simulink model "aero"  (R2024a)
settings: configuration reference "standardSILConfiguraitonParams" (kept outside this file)
undefined symbols (not defined in the file): m2ft, vehicleParams
libraries: aerolibconvert2 x5, aerolibasang x1, matrix_library x1
settings Model: Creator=GTAR  LastModifiedBy=jerem
settings ConfigSetRef: SourceName=standardSILConfiguraitonParams  SourceLocation=Base Workspace

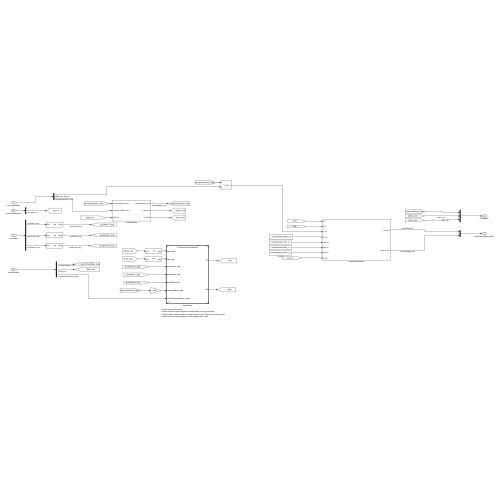
[thumbnail: Simulink's stored preview of the top-level diagram]
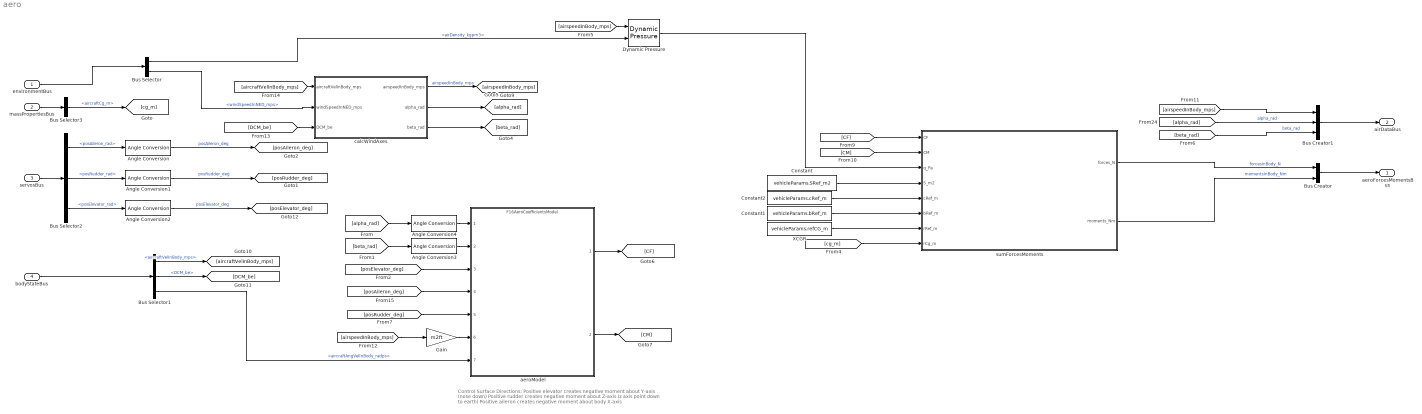
== system aero ==
  note: Control Surface Directions:
      | Positive elevator creates negative moment about Y-axis (nose down)
      | Positive rudder creates negative moment about Z-axis (z axis point down to earth)
      | Positive aileron creates negative moment about body X-axis
  environmentBus : Inport  OutDataTypeStr=Bus: EnvironmentBus
  massPropertiesBus : Inport  Port=2  OutDataTypeStr=Bus: MassPropertiesBus
  servosBus : Inport  Port=3  OutDataTypeStr=Bus: ServosBus
  bodyStateBus : Inport  Port=4  OutDataTypeStr=Bus: BodyStateBus
  Angle Conversion{,1..4} (5 alike) : aerolibconvert2/Angle Conversion  IU=rad  OU=deg
  Bus Creator : BusCreator  Inputs=2
  Bus Creator1 : BusCreator  Inputs=3
  Bus Selector : BusSelector  OutputSignals=AirEnvironment.airDensity_kgpm3,AirEnvironment.windSpeedInNED_mps
  Bus Selector1 : BusSelector  OutputSignals=aircraftVelInBody_mps,DCM_be,aircraftAngVelInBody_radps
  Bus Selector2 : BusSelector  OutputSignals=ServosF16Bus.posAileron_rad,ServosF16Bus.posRudder_rad,ServosF16Bus.posElevator_rad
  Bus Selector3 : BusSelector  OutputSignals=aircraftCg_m
  Constant : Constant  Value=vehicleParams.SRef_m2
  Constant1 : Constant  Value=vehicleParams.bRef_m
  Constant2 : Constant  Value=vehicleParams.cRef_m
  Dynamic Pressure : aerolibasang/Dynamic Pressure
  Gain : Gain  Gain=m2ft
  XCGR : Constant  Value=vehicleParams.refCG_m
  aeroModel : ModelReference  ModelNameDialog=F16AeroCoefficientsModel.slx  SimulationMode=Normal  ModelReferenceVersion=1.183
  calcWindAxes : Subsystem
  sumForcesMoments : Subsystem
  aeroForcesMomentsBus : Outport  OutDataTypeStr=Bus: ComponentForcesMomentsBus
  airDataBus : Outport  Port=2  OutDataTypeStr=Bus: AirData
  wires:
  Bus Creator/1 -> aeroForcesMomentsBus/1
  sumForcesMoments/1(forces_N) -> Bus Creator/1  "forcesInBody_N"
  sumForcesMoments/2(moments_Nm) -> Bus Creator/2  "momentsInBody_Nm"
  [cg_m] -> sumForcesMoments/8(rCg_m)
  Dynamic Pressure/1 -> sumForcesMoments/3(q_Pa)
  Angle Conversion/1 -> [posAileron_deg]  "posAileron_deg"
  environmentBus/1 -> Bus Selector/1
  Bus Selector/1 -> Dynamic Pressure/2  "<airDensity_kgpm3>"
  Bus Selector/2 -> calcWindAxes/2(windSpeedInNED_mps)  "<windSpeedInNED_mps>"
  servosBus/1 -> Bus Selector2/1
  Bus Selector2/1 -> Angle Conversion/1  "<posAileron_rad>"
  massPropertiesBus/1 -> Bus Selector3/1
  Bus Selector3/1 -> [cg_m]  "<aircraftCg_m>"
  bodyStateBus/1 -> Bus Selector1/1
  Bus Creator1/1 -> airDataBus/1
  Bus Selector2/2 -> Angle Conversion1/1  "<posRudder_rad>"
  Bus Selector2/3 -> Angle Conversion2/1  "<posElevator_rad>"
  Angle Conversion1/1 -> [posRudder_deg]  "posRudder_deg"
  Angle Conversion2/1 -> [posElevator_deg]  "posElevator_deg"
  [beta_rad] -> Bus Creator1/3  "beta_rad"
  [alpha_rad] -> Bus Creator1/2  "alpha_rad"
  [alpha_rad] -> Angle Conversion4/1
  [posElevator_deg] -> aeroModel/3
  [posAileron_deg] -> aeroModel/4
  aeroModel/1 -> [CF]
  aeroModel/2 -> [CM]
  [CF] -> sumForcesMoments/1(CF)
  [CM] -> sumForcesMoments/2(CM)
  calcWindAxes/1(airspeedInBody_mps) -> [airspeedInBody_mps]  "airspeedInBody_mps"
  [airspeedInBody_mps] -> Dynamic Pressure/1
  [airspeedInBody_mps] -> Bus Creator1/1
  [airspeedInBody_mps] -> Gain/1
  Bus Selector1/3 -> aeroModel/7  "<aircraftAngVelInBody_radps>"
  [beta_rad] -> Angle Conversion3/1
  Angle Conversion3/1 -> aeroModel/2
  Angle Conversion4/1 -> aeroModel/1
  Bus Selector1/1 -> [aircraftVelInBody_mps]  "<aircraftVelInBody_mps>"
  Bus Selector1/2 -> [DCM_be]  "<DCM_be>"
  [DCM_be] -> calcWindAxes/3(DCM_be)
  [aircraftVelInBody_mps] -> calcWindAxes/1(aircraftVelInBody_mps)
  [posRudder_deg] -> aeroModel/5
  Gain/1 -> aeroModel/6
  Constant2/1 -> sumForcesMoments/5(cRef_m)
  XCGR/1 -> sumForcesMoments/7(rRef_m)
  Constant1/1 -> sumForcesMoments/6(bRef_m)
  Constant/1 -> sumForcesMoments/4(S_m2)
  calcWindAxes/2(alpha_rad) -> [alpha_rad]
  calcWindAxes/3(beta_rad) -> [beta_rad]

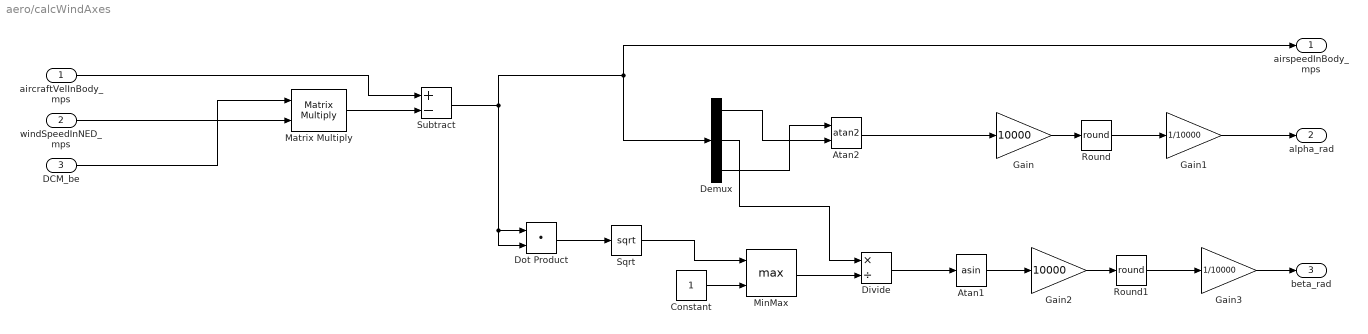
== system aero/calcWindAxes ==
  aircraftVelInBody_mps : Inport
  windSpeedInNED_mps : Inport  Port=2
  DCM_be : Inport  Port=3
  Atan1 : Trigonometry  Operator=asin
  Atan2 : Trigonometry  Operator=atan2
  Constant : Constant
  Demux : Demux  Outputs=3
  Divide : Product  Inputs=*/
  Dot Product : DotProduct  OutDataTypeStr=Inherit: Inherit via internal rule
  Gain : Gain  Gain=10000
  Gain1 : Gain  Gain=1/10000
  Gain2 : Gain  Gain=10000
  Gain3 : Gain  Gain=1/10000
  Matrix Multiply : Product  Multiplication=Matrix(*)
  MinMax : MinMax  Function=max  Inputs=2
  Round : Rounding  Operator=round
  Round1 : Rounding  Operator=round
  Sqrt : Sqrt
  Subtract : Sum  Inputs=+-
  airspeedInBody_mps : Outport
  alpha_rad : Outport  Port=2
  beta_rad : Outport  Port=3
  wires:
  DCM_be/1 -> Matrix Multiply/1
  windSpeedInNED_mps/1 -> Matrix Multiply/2
  Matrix Multiply/1 -> Subtract/2
  aircraftVelInBody_mps/1 -> Subtract/1
  Subtract/1 -> Dot Product/2, Dot Product/1, Demux/1, airspeedInBody_mps/1
  Dot Product/1 -> Sqrt/1
  Constant/1 -> MinMax/2
  Sqrt/1 -> MinMax/1
  MinMax/1 -> Divide/2
  Demux/2 -> Divide/1
  Divide/1 -> Atan1/1
  Demux/1 -> Atan2/2
  Demux/3 -> Atan2/1
  Atan2/1 -> Gain/1
  Gain/1 -> Round/1
  Round/1 -> Gain1/1
  Gain1/1 -> alpha_rad/1
  Round1/1 -> Gain3/1
  Gain2/1 -> Round1/1
  Atan1/1 -> Gain2/1
  Gain3/1 -> beta_rad/1

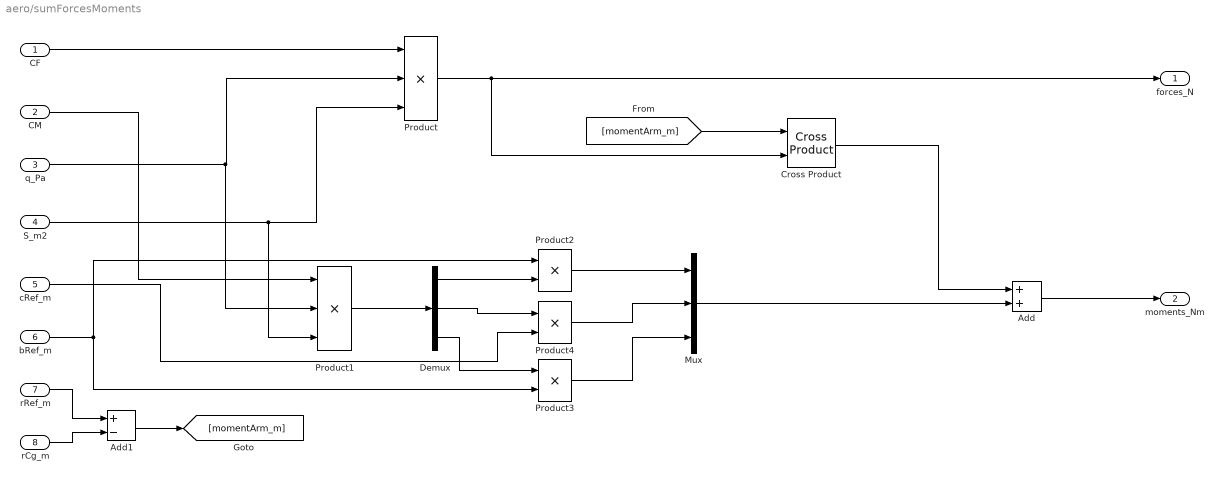
== system aero/sumForcesMoments ==
  CF : Inport
  CM : Inport  Port=2
  q_Pa : Inport  Port=3
  S_m2 : Inport  Port=4
  cRef_m : Inport  Port=5
  bRef_m : Inport  Port=6
  rRef_m : Inport  Port=7
  rCg_m : Inport  Port=8
  Add : Sum
  Add1 : Sum  Inputs=+-
  Cross Product : matrix_library/Cross Product
  Demux : Demux  Outputs=3
  Mux : Mux  Inputs=3
  Product : Product  Inputs=3
  Product1 : Product  Inputs=3
  Product2 : Product
  Product3 : Product
  Product4 : Product
  forces_N : Outport
  moments_Nm : Outport  Port=2
  wires:
  Product/1 -> Cross Product/2, forces_N/1
  CF/1 -> Product/1
  q_Pa/1 -> Product1/2, Product/2
  S_m2/1 -> Product1/3, Product/3
  CM/1 -> Product1/1
  Product1/1 -> Demux/1
  Demux/1 -> Product2/2
  bRef_m/1 -> Product3/2, Product2/1
  Product2/1 -> Mux/1
  Demux/3 -> Product3/1
  Demux/2 -> Product4/1
  cRef_m/1 -> Product4/2
  Product4/1 -> Mux/2
  Product3/1 -> Mux/3
  Mux/1 -> Add/2
  Cross Product/1 -> Add/1
  Add/1 -> moments_Nm/1
  rRef_m/1 -> Add1/1
  rCg_m/1 -> Add1/2
  Add1/1 -> [momentArm_m]
  [momentArm_m] -> Cross Product/1
